simulink model "Modello_con_integratore"  (R2019b)
settings: Solver=FixedStepAuto  StartTime=0.0  StopTime=10.0  FixedStep=Ts/10  RelTol=1e-8  AbsTol=1e-9
values from neighbouring files (symbols this model uses):
  Festar1 = F1-L1*[1 0 0]    [TestDIST_EFFECT_DCmotor.m]
  Gestar1 = [G1 L1]    [TestDIST_EFFECT_DCmotor.m]
  KK = dlqr(Fs,Gs,Q,R)    [TestDIST_EFFECT_DCmotor.m]
  Ts = 0.001    [TestDIST_EFFECT_DCmotor.m]
libraries: simulink x2
settings Model: Creator=oboe  LastModifiedBy=Luca
settings SolverCC: AutoScaleAbsTol=off
settings DataIOCC: ReturnWorkspaceOutputs=off
settings DebuggingCC: ArithmeticOperatorsInVariantConditions=warning
settings SFSimCC: SimUseLocalCustomCode=off  CustomCodeUndefinedFunction=UseInterfaceOnly
settings RTWCC: RTWUseLocalCustomCode=off
settings CodeAppCC: StateflowObjectComments=on

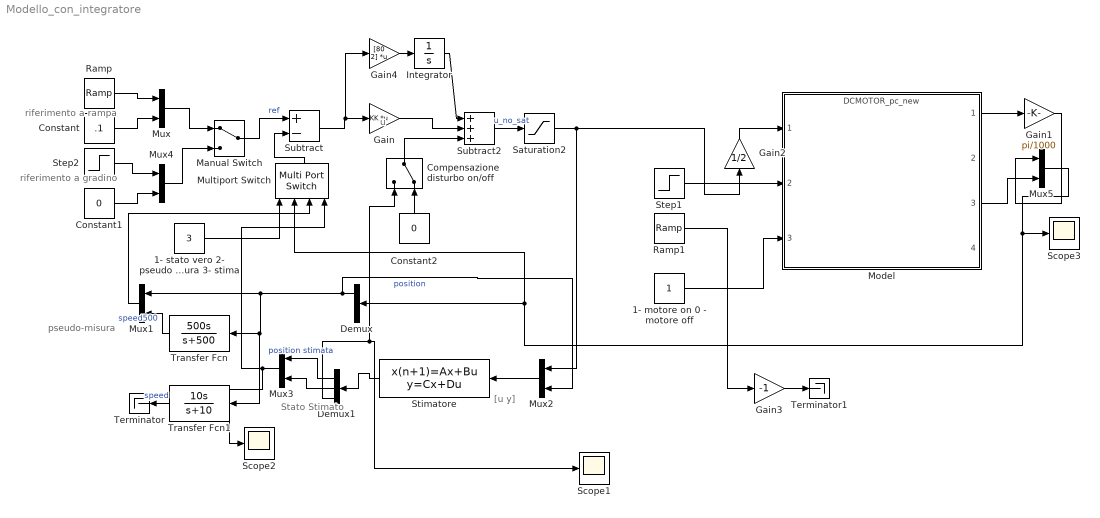
== system Modello_con_integratore ==
  note: riferimento
      | a rampa
  note: pseudo-misura
  note: [u
      | y]
  note: Stato
      | Stimato
  note: u
  note: riferimento
      | a gradino
  1- motore on 0 - motore off : Constant
  1- stato vero 2- pseudo misura 3- stima : Constant  Value=3
  Compensazione disturbo on/off : ManualSwitch  CurrentSetting=0
  Constant : Constant  Value=.1
  Constant1 : Constant  Value=0
  Constant2 : Constant  Value=0
  Demux : Demux  Outputs=2
  Demux1 : Demux  Outputs=3
  Gain : Gain  Gain=KK  Multiplication=Matrix(K*u)
  Gain1 : Gain  Gain=pi/1000
  Gain2 : Gain  Gain=1/2
  Gain3 : Gain  Gain=-1
  Gain4 : Gain  Gain=[80 2]  Multiplication=Matrix(K*u)
  Integrator : Integrator
  Manual Switch : ManualSwitch
  Model : ModelReference  ModelNameDialog=DCMOTOR_pc_new.slxp  ModelReferenceVersion=1.21  CopyOfModelProtected=on
  Multiport Switch : MultiPortSwitch
  Mux{,1..5} (6 alike) : Mux  Inputs=2
  Ramp : simulink/Sources/Ramp  slope=0.1  start=0  InitialOutput=0
  Ramp1 : simulink/Sources/Ramp  slope=.05  start=3  InitialOutput=0
  Saturation2 : Saturate  UpperLimit=6  LowerLimit=-6
  Scope1 : Scope
  Scope2 : Scope
  Scope3 : Scope
  Step1 : Step  Time=3  After=.1  SampleTime=0
  Step2 : Step  SampleTime=0
  Stimatore : DiscreteStateSpace  A=Festar1  B=Gestar1  C=eye(3)  D=[0 0; 0 0 ; 0 0]  InitialCondition=[0 0 0]'  SampleTime=Ts
  Subtract : Sum  Inputs=+-
  Subtract2 : Sum  Inputs=+++
  Terminator : Terminator
  Terminator1 : Terminator
  Transfer Fcn : TransferFcn  Numerator=[500 0]  Denominator=[1 500]
  Transfer Fcn1 : TransferFcn  Numerator=[10 0]  Denominator=[1 10]
  wires:
  Mux5/1 -> Demux/1, Multiport Switch/2, Scope3/1
  Subtract/1 -> Gain4/1, Gain/1
  Constant/1 -> Mux/2
  Ramp/1 -> Mux/1
  Demux/1 -> Mux2/2, Transfer Fcn1/1, Transfer Fcn/1, Mux1/1  "position"
  Transfer Fcn/1 -> Mux1/2  "speed500"
  Mux2/1 -> Stimatore/1
  Mux1/1 -> Multiport Switch/3
  1- stato vero 2- pseudo misura 3- stima/1 -> Multiport Switch/1
  Multiport Switch/1 -> Subtract/2
  Gain/1 -> Subtract2/2
  Demux1/1 -> Mux3/1  "position stimata"
  Mux3/1 -> Scope2/1, Multiport Switch/4
  Stimatore/1 -> Demux1/1
  Constant1/1 -> Mux4/2
  Step2/1 -> Mux4/1
  Manual Switch/1 -> Subtract/1  "ref"
  Mux/1 -> Manual Switch/1
  Mux4/1 -> Manual Switch/2
  Demux1/2 -> Mux3/2
  Demux1/3 -> Scope1/1, Compensazione disturbo on/off/1
  Compensazione disturbo on/off/1 -> Subtract2/3
  Constant2/1 -> Compensazione disturbo on/off/2
  Subtract2/1 -> Saturation2/1  "u_no_sat"
  Model/3 -> Mux5/2
  Gain2/1 -> Model/1
  1- motore on 0 - motore off/1 -> Model/3
  Gain1/1 -> Mux5/1
  Saturation2/1 -> Mux2/1, Gain2/1
  Step1/1 -> Model/2
  Model/1 -> Gain1/1
  Transfer Fcn1/1 -> Terminator/1  "speed"
  Ramp1/1 -> Gain3/1
  Gain3/1 -> Terminator1/1
  Gain4/1 -> Integrator/1
  Integrator/1 -> Subtract2/1
